simulink model "PEMFC_cEGR_Core_Physical_v01"  (R2025b)
settings: Solver=VariableStepAuto  StartTime=0.0  StopTime=500  RelTol=1e-3
PreLoadFcn:
  | addpath('D:\matlab2025b\toolbox\physmod\fluids\supporting_files\example_libraries'); addpath('E:\agentwork_pemfc_cEGR_0519\04_Simulink物理网络模型\02_参数'); P_pemfc_cEGR = PEMFC_cEGR_params_v01();
InitFcn:
  | addpath('D:\matlab2025b\toolbox\physmod\fluids\supporting_files\example_libraries'); addpath('E:\agentwork_pemfc_cEGR_0519\04_Simulink物理网络模型\02_参数'); P_pemfc_cEGR = PEMFC_cEGR_params_v01();
undefined symbols (not defined in the file): P_pemfc_cEGR
libraries: FuelCell_lib x17, nesl_utility x13, fl_lib x8
(part 3 of 3)

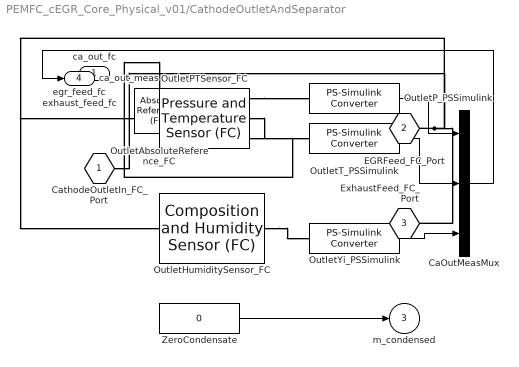
== system PEMFC_cEGR_Core_Physical_v01/CathodeOutletAndSeparator ==
  ca_out_fc : Inport
  CaOutMeasMux : Mux  Inputs=3
  OutletAbsoluteReference_FC : FuelCell_lib/elements/Absolute Reference (FC)
      settings: InternalSimscapePortConfiguration="{\"Bottom\":[],\"Left\":[{\"id\":\"A\",\"label\":\"\",\"type\":\"FuelCell.FuelCell\"}],\"Right\":[],\"Top\":[]}"
  OutletHumiditySensor_FC : FuelCell_lib/sensors/Composition and Humidity Sensor (FC)
      settings: InternalSimscapePortConfiguration="{\"Bottom\":[],\"Left\":[{\"id\":\"A\",\"label\":\"A\",\"type\":\"FuelCell.FuelCell\"}],\"Right\":[{\"id\":\"x_i\",\"label\":\"x_i\",\"type\":\"output\"},{\"id\":\"y_i\",\"label\":\"y_i\",\"type\":\"output\"},{\"id\":\"W\",\"label\":\"W\",\"type\":\"output\"}],\"Top\":[]}"
  OutletPTSensor_FC : FuelCell_lib/sensors/Pressure and Temperature Sensor (FC)
      settings: InternalSimscapePortConfiguration="{\"Bottom\":[],\"Left\":[{\"id\":\"A\",\"label\":\"A\",\"type\":\"FuelCell.FuelCell\"}],\"Right\":[{\"id\":\"P\",\"label\":\"P\",\"type\":\"output\"},{\"id\":\"T\",\"label\":\"T\",\"type\":\"output\"},{\"id\":\"B\",\"label\":\"B\",\"type\":\"FuelCell.FuelCell\"}],\"Top\":[]}"
  OutletP_PSSimulink : nesl_utility/PS-Simulink Converter  PhysicalDomain=network_engine_domain  SubClassName=ps_output  LeftPortType=input  RightPortType=output  PseudoPeriodic=off  Frequencies=[]  VectorFormat=inherit  Unit=inherit  AffineConversion=off
  OutletT_PSSimulink : nesl_utility/PS-Simulink Converter  PhysicalDomain=network_engine_domain  SubClassName=ps_output  LeftPortType=input  RightPortType=output  PseudoPeriodic=off  Frequencies=[]  VectorFormat=inherit  Unit=inherit  AffineConversion=off
  OutletYi_PSSimulink : nesl_utility/PS-Simulink Converter  PhysicalDomain=network_engine_domain  SubClassName=ps_output  LeftPortType=input  RightPortType=output  PseudoPeriodic=off  Frequencies=[]  VectorFormat=inherit  Unit=inherit  AffineConversion=off
  ZeroCondensate : Constant  Value=0
  CathodeOutletIn_FC_Port : PMIOPort  Side=Left
  EGRFeed_FC_Port : PMIOPort  Port=2  Side=Right
  ExhaustFeed_FC_Port : PMIOPort  Port=3  Side=Right
  egr_feed_fc : Outport
  exhaust_feed_fc : Outport  Port=2
  m_condensed : Outport  Port=3
  ca_out_meas : Outport  Port=4
  wires:
  ZeroCondensate/1 -> m_condensed/1
  OutletP_PSSimulink/1 -> CaOutMeasMux/1
  OutletT_PSSimulink/1 -> CaOutMeasMux/2
  OutletYi_PSSimulink/1 -> CaOutMeasMux/3
  CaOutMeasMux/1 -> ca_out_meas/1
  connections:
  OutletPTSensor_FC/RConn3 -- OutletAbsoluteReference_FC/LConn1
  OutletPTSensor_FC/RConn1 -- OutletP_PSSimulink/LConn1
  OutletPTSensor_FC/RConn2 -- OutletT_PSSimulink/LConn1
  OutletHumiditySensor_FC/RConn2 -- OutletYi_PSSimulink/LConn1
  EGRFeed_FC_Port/RConn1 -- CathodeOutletIn_FC_Port/RConn1 -- ExhaustFeed_FC_Port/RConn1 -- OutletPTSensor_FC/LConn1 -- OutletHumiditySensor_FC/LConn1

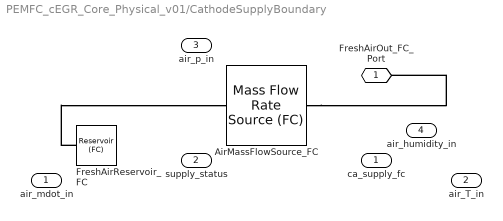
== system PEMFC_cEGR_Core_Physical_v01/CathodeSupplyBoundary ==
  air_mdot_in : Inport
  air_T_in : Inport  Port=2
  air_p_in : Inport  Port=3
  air_humidity_in : Inport  Port=4
  AirMassFlowSource_FC : FuelCell_lib/sources/Mass Flow Rate Source (FC)  source_type=foundation.enum.constant_controlled.constant  flow_rate=6e-3 kg/s  power_spec=foundation.enum.power_spec.none  area_A=0.01 m^2  area_B=0.01 m^2  mdot_A_specify=off  mdot_A_priority=None  mdot_A=0.1 kg/s  mdot_A_nominal_specify=off  mdot_A_nominal_value=1  mdot_A_nominal_unit=kg/s  mdot_B_specify=off  mdot_B_priority=None  mdot_B=0.1 kg/s  mdot_B_nominal_specify=off  mdot_B_nominal_value=1  mdot_B_nominal_unit=kg/s  phi_A_specify=off  phi_A_priority=None  phi_A=0 J/s  phi_A_nominal_specify=off  phi_A_nominal_value=1  phi_A_nominal_unit=J/s  phi_B_specify=off  phi_B_priority=None  phi_B=0 J/s  phi_B_nominal_specify=off  phi_B_nominal_value=1  phi_B_nominal_unit=J/s  mdot_A_i_specify=off  mdot_A_i_priority=None  mdot_A_i=[0; 0; 0; 0] kg/s  mdot_A_i_nominal_specify=off  mdot_A_i_nominal_value=1  mdot_A_i_nominal_unit=kg/s  mdot_B_i_specify=off  mdot_B_i_priority=None  mdot_B_i=[0; 0; 0; 0] kg/s  mdot_B_i_nominal_specify=off  mdot_B_i_nominal_value=1  mdot_B_i_nominal_unit=kg/s
      settings: InternalSimscapePortConfiguration="{\"Bottom\":[],\"Left\":[{\"id\":\"A\",\"label\":\"A\",\"type\":\"FuelCell.FuelCell\"}],\"Right\":[{\"id\":\"B\",\"label\":\"B\",\"type\":\"FuelCell.FuelCell\"}],\"Top\":[]}"
  FreshAirReservoir_FC : FuelCell_lib/elements/Reservoir (FC)  constCond=true  p0=150e3 Pa  T0=333.15 K  comp=FuelCell.enum.Composition.Mole  y0=[0.77; 0.21; 0; 0.02]  x0=[0.75; 0.23; 0; 0.02]  area=0.01 m^2
      settings: InternalSimscapePortConfiguration="{\"Bottom\":[],\"Left\":[],\"Right\":[],\"Top\":[{\"id\":\"A\",\"label\":\"A\",\"type\":\"FuelCell.FuelCell\"}]}"
  FreshAirOut_FC_Port : PMIOPort  Side=Left
  ca_supply_fc : Outport
  supply_status : Outport  Port=2
  connections:
  AirMassFlowSource_FC/RConn1 -- FreshAirOut_FC_Port/RConn1
  FreshAirReservoir_FC/LConn1 -- AirMassFlowSource_FC/LConn1

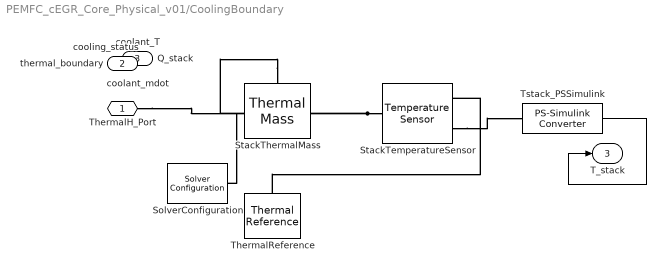
== system PEMFC_cEGR_Core_Physical_v01/CoolingBoundary ==
  coolant_T : Inport
  coolant_mdot : Inport  Port=2
  Q_stack : Inport  Port=3
  SolverConfiguration : nesl_utility/Solver Configuration  PhysicalDomain=network_engine_domain  SubClassName=solver  LeftPortType=input  RightPortType=generic  Tones=[]  Harmonics=[]  SimulateNoise=off  Profile=off  UseLocalSampling=off  EnableSwitchedLinearOptims=on  FrequencyDomain=off  UseCCode=off  RelTol=0.001  AbsTol=0.001  MinStep=1e-09  ToWorkspace=off  RevertToSquareIcSolve=off  NumHomotopyIterations=100  PhasorMode=off  PhasorModeNumHarmonics=1  ConsistencySolver=NEWTON_XTOL_AFTER_FTOL  IndexReductionMethod=DerivativeReplacement  DoDC=off  ResidualTolerance=1e-09  ConsistencyTolSource=GLOBAL  ConsistencyAbsTol=0.001  ConsistencyRelTol=0.001  ConsistencyTolFactor=0.001  UseLocalSolver=off  LocalSolverChoice=NE_BACKWARD_EULER_ADVANCER  ResolveIndetEquations=on  FunctionEvalNumThread=1  LocalSolverSampleTime=0.001  DoFixedCost=off  MaxNonlinIter=3  MaxModeIter=2  ComputeImpulses=off  ImpulseIterations=2  LinearAlgebra=auto  LinearAlgebraNumThread=0  EquationFormulation=NE_TIME_EF  DelaysMemoryBudget=1024  AutomaticFiltering=on  FilteringTimeConstant=0.001  PartitionStorageMethod=AS_NEEDED  PartitionMemoryBudget=1024  PartitionMethod=ROBUST  MultibodyUseLocalSolver=off  MultibodyLocalSolverChoice=ODE1  MultibodyLocalSolverSampleTime=0.001
  StackTemperatureSensor : fl_lib/Thermal/Thermal Sensors/Temperature Sensor  temperature_measure=foundation.enum.MeasurementReference.difference
  StackThermalMass : fl_lib/Thermal/Thermal Elements/Thermal Mass  mass_type=foundation.enum.constant_variable.constant  mass=1 kg  sp_heat=447 J/(K*kg)  mass_min=1e-6 kg  num_ports=foundation.enum.numPorts2.one  m_specify=off  m_priority=High  m=1 kg  m_nominal_specify=off  m_nominal_value=1  m_nominal_unit=kg  T_specify=off  T_priority=High  T=300 K  T_nominal_specify=off  T_nominal_value=1  T_nominal_unit=K  Q_specify=off  Q_priority=None  Q=0 W  Q_nominal_specify=off  Q_nominal_value=1  Q_nominal_unit=W
  ThermalReference : fl_lib/Thermal/Thermal Elements/Thermal Reference
  Tstack_PSSimulink : nesl_utility/PS-Simulink Converter  PhysicalDomain=network_engine_domain  SubClassName=ps_output  LeftPortType=input  RightPortType=output  PseudoPeriodic=off  Frequencies=[]  VectorFormat=inherit  Unit=inherit  AffineConversion=off
  ThermalH_Port : PMIOPort  Side=Left
  thermal_boundary : Outport
  cooling_status : Outport  Port=2
  T_stack : Outport  Port=3
  wires:
  Tstack_PSSimulink/1 -> T_stack/1
  connections:
  StackThermalMass/LConn1 -- ThermalH_Port/RConn1 -- StackTemperatureSensor/LConn1 -- SolverConfiguration/RConn1
  ThermalReference/LConn1 -- StackTemperatureSensor/RConn1
  StackTemperatureSensor/RConn2 -- Tstack_PSSimulink/LConn1

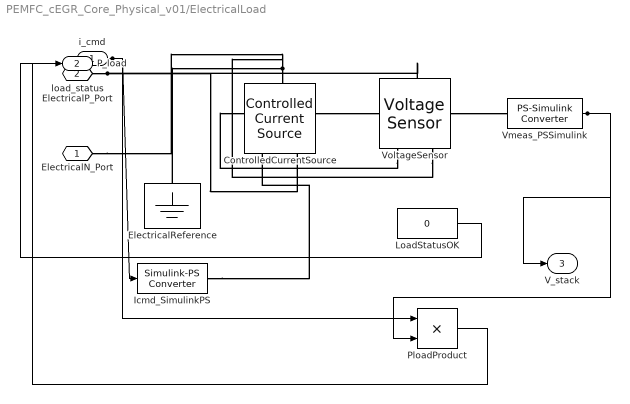
== system PEMFC_cEGR_Core_Physical_v01/ElectricalLoad ==
  i_cmd : Inport
  ControlledCurrentSource : fl_lib/Electrical/Electrical Sources/Controlled Current Source
  ElectricalReference : fl_lib/Electrical/Electrical Elements/Electrical Reference
  Icmd_SimulinkPS : nesl_utility/Simulink-PS Converter  PhysicalDomain=network_engine_domain  SubClassName=ps_input  LeftPortType=input  RightPortType=output  PseudoPeriodic=off  Frequencies=[]  NoiseDistribution=none  NoiseParameters=[]  Unit=1  AffineConversion=off  FilteringAndDerivatives=provide  SimscapeFilterOrder=1  InputFilterTimeConstant=0.001  UdotUserProvided=0
  LoadStatusOK : Constant  Value=0
  PloadProduct : Product
  Vmeas_PSSimulink : nesl_utility/PS-Simulink Converter  PhysicalDomain=network_engine_domain  SubClassName=ps_output  LeftPortType=input  RightPortType=output  PseudoPeriodic=off  Frequencies=[]  VectorFormat=inherit  Unit=inherit  AffineConversion=off
  VoltageSensor : fl_lib/Electrical/Electrical Sensors/Voltage Sensor
  ElectricalN_Port : PMIOPort  Side=Left
  ElectricalP_Port : PMIOPort  Port=2  Side=Left
  load_status : Outport
  P_load : Outport  Port=2
  V_stack : Outport  Port=3
  wires:
  i_cmd/1 -> Icmd_SimulinkPS/1, PloadProduct/1
  Vmeas_PSSimulink/1 -> PloadProduct/2, V_stack/1
  PloadProduct/1 -> P_load/1
  LoadStatusOK/1 -> load_status/1
  connections:
  Icmd_SimulinkPS/RConn1 -- ControlledCurrentSource/RConn1
  ElectricalN_Port/RConn1 -- ElectricalReference/LConn1 -- ControlledCurrentSource/LConn1 -- VoltageSensor/RConn2
  ControlledCurrentSource/RConn2 -- ElectricalP_Port/RConn1 -- VoltageSensor/LConn1
  VoltageSensor/RConn1 -- Vmeas_PSSimulink/LConn1

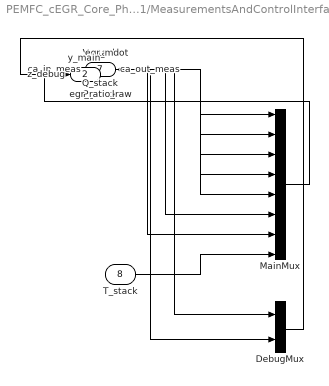
== system PEMFC_cEGR_Core_Physical_v01/MeasurementsAndControlInterface ==
  V_stack : Inport
  P_stack : Inport  Port=2
  Q_stack : Inport  Port=3
  ca_in_meas : Inport  Port=4
  ca_out_meas : Inport  Port=5
  egr_mdot : Inport  Port=6
  egr_ratio_raw : Inport  Port=7
  T_stack : Inport  Port=8
  DebugMux : Mux  Inputs=2
  MainMux : Mux  Inputs=8
  y_main : Outport
  z_debug : Outport  Port=2
  wires:
  V_stack/1 -> MainMux/1
  P_stack/1 -> MainMux/2
  Q_stack/1 -> MainMux/3
  ca_in_meas/1 -> MainMux/4
  ca_out_meas/1 -> MainMux/5
  egr_mdot/1 -> MainMux/6, DebugMux/1
  egr_ratio_raw/1 -> MainMux/7, DebugMux/2
  MainMux/1 -> y_main/1
  DebugMux/1 -> z_debug/1
  T_stack/1 -> MainMux/8

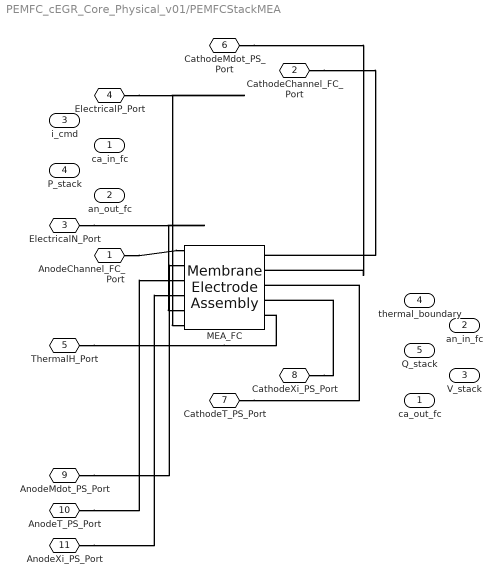
== system PEMFC_cEGR_Core_Physical_v01/PEMFCStackMEA ==
  ca_in_fc : Inport
  an_in_fc : Inport  Port=2
  i_cmd : Inport  Port=3
  thermal_boundary : Inport  Port=4
  MEA_FC : FuelCell_lib/elements/Membrane Electrode Assembly  N_cell=80  area_cell=280 cm^2  t_membrane=0.0125 cm  rtype=FuelCell.enum.ResistanceModel.Classic  RH_TLU=[0, .1, .2, .3, .4, .5, .6, .7, .8, .9, 1]  conductivity_TLU_1D=[0, .017, .035, .055, .081, .11, .15, .21, .27, .35, .45] S/cm  T_scale=1268 K  T_cond=353.15 K  T_TLU=[303.15, 353.15, 393.15] K  conductivity_TLU_2D=[0, .0093, .019, .031, .045, .063, .086, .11, .15, .2, .25; 0, .017, .035, .055, .081, .11, .15, .21, .27, .35, .45; 0, .024, .05, .08, .12, .16, .22, .3, .39, .51, .65] S/cm  io=1e-3 A/cm^2  iL=2.0 A/cm^2  alpha=0.5  rho_membrane=0.002 kg/cm^3  M_membrane=1.1 kg/mol  D_N2=2e-5 cm^2/s  Icell_specify=off  Icell_priority=None  Icell=0 A  Icell_nominal_specify=off  Icell_nominal_value=1  Icell_nominal_unit=A  HeatRxn_specify=off  HeatRxn_priority=None  HeatRxn=0 W  HeatRxn_nominal_specify=off  HeatRxn_nominal_value=1  HeatRxn_nominal_unit=W  T_stack_specify=off  T_stack_priority=None  T_stack=333.15 K  T_stack_nominal_specify=off  T_stack_nominal_value=1  T_stack_nominal_unit=K
      settings: InternalSimscapePortConfiguration="{\"Bottom\":[{\"id\":\"H\",\"label\":\"H\",\"type\":\"foundation.thermal.thermal\"}],\"Left\":[{\"id\":\"A\",\"label\":\"A\",\"type\":\"FuelCell.FuelCell\"},{\"id\":\"mdot_an\",\"label\":\"Ma\",\"type\":\"output\"},{\"id\":\"T_an\",\"label\":\"Ta\",\"type\":\"output\"},{\"id\":\"x_i_anode\",\"label\":\"xia\",\"type\":\"input\"}],\"Right\":[{\"id\":\"C\",\"label\":\"C\",\"type\":\"FuelCell.FuelCell\"},{\"id\":\"mdot_ca\",\"label\":\"Mc\",\"type\":\"output\"},{\"id\":\"T_ca\",\"label\":\"Tc\",\"type\":\"output\"},{\"id\":\"x_i_cathode\",\"label\":\"xic\",\"type\":\"input\"}],\"Top\":[{\"id\":\"n\",\"label\":\"-\",\"type\":\"foundation.electrical.electrical\"},{\"id\":\"p\",\"label\":\"+\",\"type\":\"foundation.electrical.electrical\"}]}"
  AnodeChannel_FC_Port : PMIOPort  Side=Left
  CathodeChannel_FC_Port : PMIOPort  Port=2  Side=Left
  ElectricalN_Port : PMIOPort  Port=3  Side=Left
  ElectricalP_Port : PMIOPort  Port=4  Side=Left
  ThermalH_Port : PMIOPort  Port=5  Side=Left
  CathodeMdot_PS_Port : PMIOPort  Port=6  Side=Right
  CathodeT_PS_Port : PMIOPort  Port=7  Side=Right
  CathodeXi_PS_Port : PMIOPort  Port=8  Side=Right
  AnodeMdot_PS_Port : PMIOPort  Port=9  Side=Left
  AnodeT_PS_Port : PMIOPort  Port=10  Side=Left
  AnodeXi_PS_Port : PMIOPort  Port=11  Side=Left
  ca_out_fc : Outport
  an_out_fc : Outport  Port=2
  V_stack : Outport  Port=3
  P_stack : Outport  Port=4
  Q_stack : Outport  Port=5
  connections:
  CathodeXi_PS_Port/RConn1 -- MEA_FC/RConn4
  CathodeT_PS_Port/RConn1 -- MEA_FC/RConn3
  CathodeMdot_PS_Port/RConn1 -- MEA_FC/RConn2
  ThermalH_Port/RConn1 -- MEA_FC/RConn5
  ElectricalP_Port/RConn1 -- MEA_FC/LConn6
  ElectricalN_Port/RConn1 -- MEA_FC/LConn5
  CathodeChannel_FC_Port/RConn1 -- MEA_FC/RConn1
  AnodeChannel_FC_Port/RConn1 -- MEA_FC/LConn1
  AnodeMdot_PS_Port/RConn1 -- MEA_FC/LConn2
  AnodeT_PS_Port/RConn1 -- MEA_FC/LConn3
  AnodeXi_PS_Port/RConn1 -- MEA_FC/LConn4
